simulink model "PTBS_ICE_vehicle_DCT"  (R2023b)
settings: Solver=FixedStepAuto  StartTime=0.0  StopTime=1373  FixedStep=0.002  RelTol=1e-3
model workspace (MAT data in the model file):
  Af = 4
  Cd = 0.3
  DownShiftSpeeds = [8.45 25.45 42.45 59.45 76.45 11.25 28.25 45.25 62.25 79.25 14 31 ... (20 elements, 5x4)]
  DrCycles : object (value not decoded)
  I = 5
  Kbr = 500000
  P = 32
  PedalPositions = [10 40 50 90]
  TWAIT = 5
  TimeHWFET = 765
  TimeUDDS = 1372
  TimeUS06 = 596
  UpShiftSpeeds = [11.45 28.45 45.45 62.45 79.45 14.25 31.25 48.25 65.25 82.25 17 34 ... (20 elements, 5x4)]
  axle_b = 10
  axle_k = 5000
  bevAxle_wc = 400
  bevNp = 2
  bevNs = 30
  diffRatio = 3.4
  diffRatio1 = 3.4
  engineSpeedPoints_rpm = [750 1053.57142857 1357.14285714 1660.71428571 1964.28571429 2267.85714286 2571.42857143 2875 3178.57142857 3482.14285714 3785.71428571 4089.28571429 ... (15 elements, 1x15)]
  engineTorqueMap_Nm = [0 15.0034460821 26.4289521305 37.8539339756 49.2854604964 60.7146317399 72.0173711595 77.7345012802 77.7345012802 77.7345012802 77.7345012802 77.7345012802 ... (240 elements, 16x15)]
  engineTorquePoints_Nm = [0 15 26.4285714286 37.8571428571 49.2857142857 60.7142857143 72.1428571429 83.5714285714 95 106.428571429 117.857142857 129.285714286 ... (16 elements, 1x16)]
  motorMaxTorqueNm = [500 500 500 500 500 500 416.666666667 357.142857143 312.5 277.777777778 250 227.272727273 ... (16 elements, 1x16)]
  motorSpeedRadPs = [0 40 80 120 160 200 240 280 320 360 400 440 ... (16 elements, 1x16)]
  vehicleMass = 1500
  wheelRadius = 0.35
libraries: autolibshared x3, autolibsharedcoupling x2, autolibshareddiff x1, slpidlib x1, autolibsharedmappedengines x1, autolibtransdct x1
(part 5 of 5)

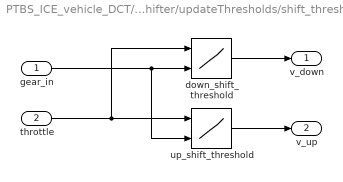
== system PTBS_ICE_vehicle_DCT/VCU/Shifter/updateThresholds/shift_threshold ==
  gear_in : Inport
  throttle : Inport  Port=2
  down_shift_threshold : Lookup2D  RowIndex=PedalPositions  ColumnIndex=[2:6]  Table=DownShiftSpeeds'  SaturateOnIntegerOverflow=off
  up_shift_threshold : Lookup2D  RowIndex=PedalPositions  ColumnIndex=[1:5]  Table=UpShiftSpeeds'  SaturateOnIntegerOverflow=off
  v_down : Outport  VectorParamsAs1DForOutWhenUnconnected=off
  v_up : Outport  Port=2  VectorParamsAs1DForOutWhenUnconnected=off
  wires:
  up_shift_threshold/1 -> v_up/1
  down_shift_threshold/1 -> v_down/1
  throttle/1 -> up_shift_threshold/1, down_shift_threshold/1
  gear_in/1 -> up_shift_threshold/2, down_shift_threshold/2

== stateflow chart PTBS_ICE_vehicle_DCT/VCU/Shifter ==
  settings: updateMethod=DISCRETE  sampleTime=0.05
  state ShiftControl [parallel]
    during:
    [v_down,v_up]=updateThresholds(gear,throttle);
    settings: executionOrder=1
    state Steady
    state Downshifting
    state Upshifting
    (default) -> Steady
    Steady -> Downshifting [order 2] : [v < v_down]
    Steady -> Upshifting [order 1] : [v > v_up]
    Downshifting -> Steady [order 2] : after(3,tick)
        | [v <= v_down]
        | {send(DOWN,GearControl)}
    Downshifting -> Steady [order 1] : [v > v_down]
    Upshifting -> Steady [order 1] : after(3,tick)
        | [v >= v_up]
        | {send(UP,GearControl)}
    Upshifting -> Steady [order 2] : [v < v_up]
  state GearControl [parallel]
    settings: executionOrder=2
    state Gear_2
      entry:
      gear = 2;
    state Gear_4
      en: gear = 4;
    state Gear_5
      en: gear = 5;
    state Gear_6
      en: gear = 6;
    state Gear_3
      en: gear = 3;
    state Gear_1
      entry:
      gear = 1;
    (default) -> Gear_1
    Gear_5 -> Gear_6 [order 2] : UP
    Gear_2 -> Gear_3 [order 1] : UP
    Gear_3 -> Gear_4 [order 1] : UP
    Gear_1 -> Gear_2 : UP
    Gear_4 -> Gear_5 [order 2] : UP
    Gear_5 -> Gear_4 [order 1] : DOWN
    Gear_2 -> Gear_1 [order 2] : DOWN
    Gear_3 -> Gear_2 [order 2] : DOWN
    Gear_6 -> Gear_5 : DOWN
    Gear_4 -> Gear_3 [order 1] : DOWN
  state [downTH,upTH] = updateThresholds(gearNum,throttleVal) [function]
  data: gearNum function_input double size=1; throttleVal function_input double size=1; downTH function_output; upTH function_output; v_up local double; v_down local double; gear output double; throttle input double; v input double
  events: UP local FUNCTION_CALL_EVENT; DOWN local FUNCTION_CALL_EVENT
